simulink model "Ejercicio_3_c"  (R2023a)
settings: Solver=VariableStepAuto  StartTime=0.0  StopTime=5  RelTol=1e-3
values from neighbouring files (symbols this model uses):
  A = [0 1; -k/m 0]    [Ejercicio_3.m]
  B = [0; 1/m]    [Ejercicio_3.m]
  g0 = utilsMati.realim_VE.factorEscala(A,B,C,K)    [Ejercicio_3.m]
  K = 2    [Ejercicio_2.m]    (also in Ejercicio_3.m = acker(A, B, PLC_VE))
settings Model: Creator=Mati  LastModifiedBy=Mati

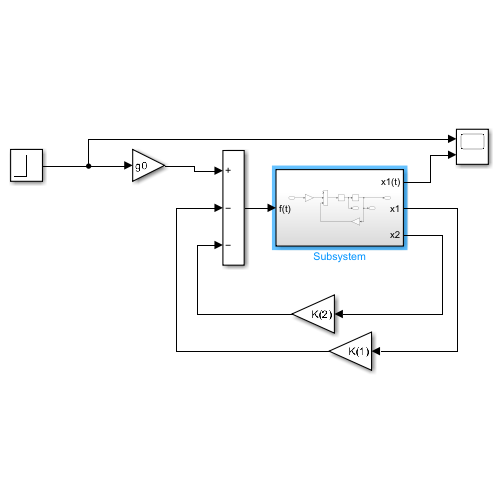
[thumbnail: Simulink's stored preview of the top-level diagram]
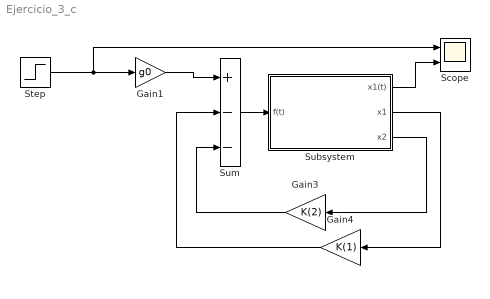
== system Ejercicio_3_c ==
  Gain1 : Gain  Gain=g0
  Gain3 : Gain  Gain=K(2)
  Gain4 : Gain  Gain=K(1)
  Scope : Scope  NumInputPorts=2
  Step : Step  SampleTime=0
  Subsystem : Subsystem
  Sum : Sum  Inputs=+--
  wires:
  Sum/1 -> Subsystem/1(f(t))
  Subsystem/1(x1(t)) -> Scope/2
  Gain3/1 -> Sum/3
  Gain4/1 -> Sum/2
  Subsystem/3(x2) -> Gain3/1
  Subsystem/2(x1) -> Gain4/1
  Step/1 -> Scope/1, Gain1/1
  Gain1/1 -> Sum/1

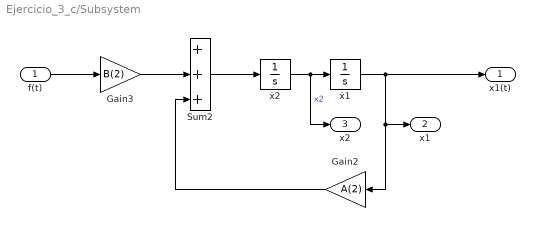
== system Ejercicio_3_c/Subsystem ==
  f(t) : Inport
  Gain2 : Gain  Gain=A(2)
  Gain3 : Gain  Gain=B(2)
  Sum2 : Sum  Inputs=+++
  ẋ1 : Integrator
  ẋ2 : Integrator
  x1(t) : Outport
  x1 : Outport  Port=2
  x2 : Outport  Port=3
  wires:
  ẋ2/1 -> x2/1, ẋ1/1  "x2"
  ẋ1/1 -> x1(t)/1, x1/1, Gain2/1
  f(t)/1 -> Gain3/1
  Gain3/1 -> Sum2/2
  Gain2/1 -> Sum2/3
  Sum2/1 -> ẋ2/1
